simulink model "aircraft"  (R2018a)
settings: Solver=FixedStepAuto  StartTime=0.0  StopTime=10.0  FixedStep=0.02  RelTol=1e-3
model workspace (MAT data in the model file):
  Beta = 426.4352
  Gamma = 0.01
  Ka = 0.677
  Kf = -1.746
  Ki = -3.864
  Kq = 0.8156
  Md = -6.8847
  Mq = -0.6571
  Mw = -0.00592
  Sa = 0.005236
  Swg = 3
  Ta = 0.05
  Tal = 0.3959
  Ts = 0.1
  Uo = 689.4
  Vto = 690.4
  W1 = 2.971
  W2 = 4.144
  Wa = 10
  Zd = -63.9979
  Zw = -0.6385
  a = 2.5348
  b = 64.13
  cmdgain = 0.0349095447273
  g = 32.2
undefined symbols (not defined in the file): a_max, a_min, adva_max, adva_min, x_ini, x_max, x_min
libraries: simulink x2
settings Model: TunableVars=a_max,a_min,adva_max,adva_min,x_ini,x_max,x_min  TunableVarsStorageClass=Auto,Auto,Auto,Auto,Auto,Auto,Auto  TunableVarsTypeQualifier=,,,,,,  OrderedModelArguments=off  Creator=hjzsj  LastModifiedBy=Jet
settings DataIOCC: ReturnWorkspaceOutputs=on
settings OptimizationCC: DefaultParameterBehavior=Inlined  UseDivisionForNetSlopeComputation=on  UseFloatMulNetSlope=on  PassReuseOutputArgsAs=Individual arguments  NoFixptDivByZeroProtection=on  EfficientFloat2IntCast=on  LifeSpan=1  OptimizeBlockOrder=speed  DifferentSizesBufferReuse=on
settings DebuggingCC: ParameterTunabilityLossMsg=error
settings HardwareCC: ProdLongLongMode=on
settings SFSimCC: SimUseLocalCustomCode=on  MATLABDynamicMemAlloc=off
settings RTWCC: SystemTargetFile=ert.tlc  GenCodeOnly=on  TemplateMakefile=ert_default_tmf  PostCodeGenCommand=mat2json  RTWUseLocalCustomCode=on  TargetLang=C++
settings CodeAppCC: ForceParamTrailComments=on  IgnoreCustomStorageClasses=off  OperatorAnnotations=on  SimulinkDataObjDesc=on  SFDataObjDesc=on  CustomSymbolStrGlobalVar=rt$N$M  CustomSymbolStrType=$N$M  CustomSymbolStrFcn=$N$M$F  CustomSymbolStrMacro=$N$M  InsertBlockDesc=on
settings ERTTargetCC: TargetLangStandard=C++03 (ISO)  GenerateSampleERTMain=on  CombineSignalStateStructs=on  MultiInstanceERTCode=on  CodeInterfacePackaging=C++ class  SupportComplex=off  SupportContinuousTime=on  InlinedParameterPlacement=NonHierarchical  RootIOFormat=Structure reference  ERTCustomFileTemplate=example_file_process.tlc  ERTFilePackagingFormat=CompactWithDataFile

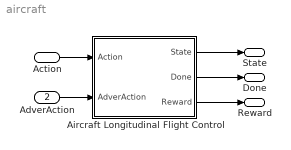
== system aircraft ==
  Action : Inport
  AdverAction : Inport  Port=2
  Aircraft Longitudinal Flight Control : Subsystem
  State : Outport  VectorParamsAs1DForOutWhenUnconnected=on
  Done : Outport  Port=2  VectorParamsAs1DForOutWhenUnconnected=on
  Reward : Outport  Port=3  VectorParamsAs1DForOutWhenUnconnected=on
  wires:
  Aircraft Longitudinal Flight Control/1(State) -> State/1
  Aircraft Longitudinal Flight Control/2(Done) -> Done/1
  Action/1 -> Aircraft Longitudinal Flight Control/1(Action)
  Aircraft Longitudinal Flight Control/3(Reward) -> Reward/1
  AdverAction/1 -> Aircraft Longitudinal Flight Control/2(AdverAction)

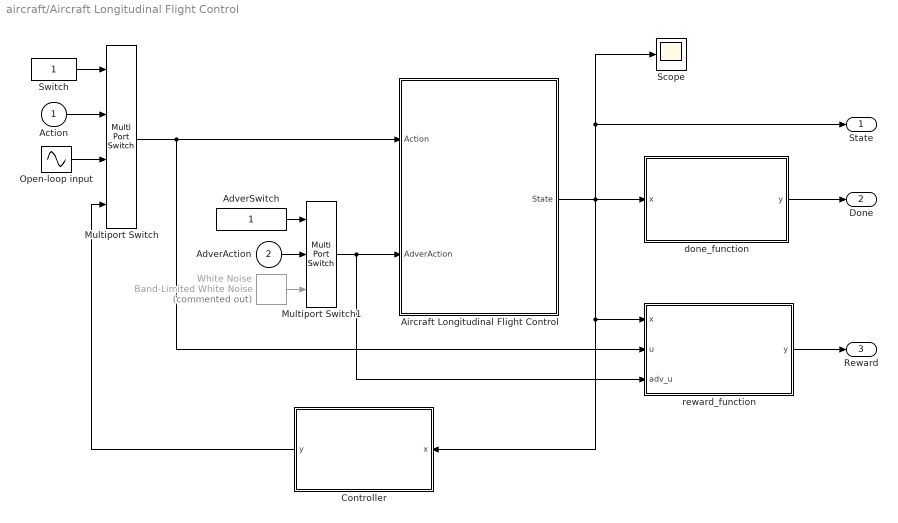
== system aircraft/Aircraft Longitudinal Flight Control ==
  Action : Inport
  AdverAction : Inport  Port=2
  AdverSwitch : Constant
  Aircraft Longitudinal Flight Control : Subsystem
  Controller : MATLAB Function  TreatAsAtomicUnit=on
  Multiport Switch : MultiPortSwitch
  Multiport Switch1 : MultiPortSwitch  Inputs=2
  Open-loop input : Sin  SampleTime=0
  Scope : Scope
  Switch : Constant
  White Noise : simulink/Sources/Band-Limited White Noise  Commented=on  Cov=[0.5]  Ts=0.02  seed=[23341]
  done_function : MATLAB Function  TreatAsAtomicUnit=on
  reward_function : MATLAB Function  TreatAsAtomicUnit=on
  State : Outport  VectorParamsAs1DForOutWhenUnconnected=on
  Done : Outport  Port=2  VectorParamsAs1DForOutWhenUnconnected=on
  Reward : Outport  Port=3  VectorParamsAs1DForOutWhenUnconnected=on
  wires:
  Aircraft Longitudinal Flight Control/1(State) -> Controller/1(x), reward_function/1(x), Scope/1, State/1, done_function/1(x)
  reward_function/1(y) -> Reward/1
  Open-loop input/1 -> Multiport Switch/3
  done_function/1(y) -> Done/1
  Switch/1 -> Multiport Switch/1
  Multiport Switch/1 -> reward_function/2(u), Aircraft Longitudinal Flight Control/1(Action)
  Action/1 -> Multiport Switch/2
  Controller/1(y) -> Multiport Switch/4
  Multiport Switch1/1 -> reward_function/3(adv_u), Aircraft Longitudinal Flight Control/2(AdverAction)
  AdverSwitch/1 -> Multiport Switch1/1
  White Noise/1 -> Multiport Switch1/3
  AdverAction/1 -> Multiport Switch1/2

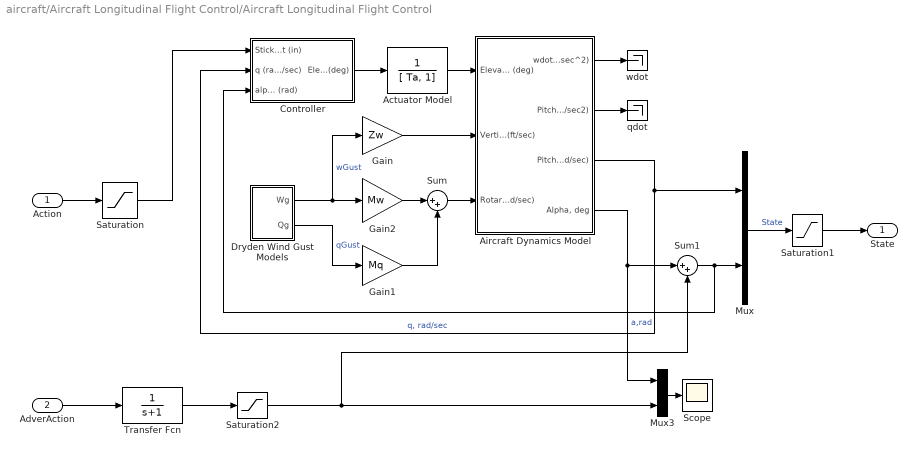
== system aircraft/Aircraft Longitudinal Flight Control/Aircraft Longitudinal Flight Control ==
  Action : Inport
  AdverAction : Inport  Port=2
  Actuator Model : TransferFcn  Denominator=[ Ta, 1]
  Aircraft Dynamics Model : Subsystem
      mask Display:
      | port_label('input',1,'\delta_{e}, deg','texmode','on');
      | port_label('input',2,'wGust, ft/sec','texmode','on');
      | port_label('input',3,'qGust, rad/sec','texmode','on');
      | port_label('output',1,'wdot, ft/sec^2','texmode','on');
      | port_label('output',2,'qdot, rad/sec^{2}','texmode','on');
      | port_label('output',3,'q, rad/sec','texmode','on');
      | port_label('output',4,'\alpha, rad','texmode','on');
  Controller : Subsystem
      mask Display:
      | port_label('input',1,'Stick, in','texmode','on');
      | port_label('input',3,'\alpha, rad','texmode','on');
      | port_label('input',2,'q, rad/sec','texmode','on');
      | port_label('output',1,'\deltacmd, deg','texmode','on');
  Dryden Wind Gust Models : Subsystem
      mask Display:
      | port_label('output',1,'wg','texmode','on');
      | port_label('output',2,'qg','texmode','on');
  Gain : Gain  Gain=Zw  SaturateOnIntegerOverflow=on  OutDataTypeStr=Inherit: Same as input  ParamDataTypeStr=Inherit: Same as input
  Gain1 : Gain  Gain=Mq  SaturateOnIntegerOverflow=on  OutDataTypeStr=Inherit: Same as input  ParamDataTypeStr=Inherit: Same as input
  Gain2 : Gain  Gain=Mw  SaturateOnIntegerOverflow=on  OutDataTypeStr=Inherit: Same as input  ParamDataTypeStr=Inherit: Same as input
  Mux : Mux  Inputs=2
  Mux3 : Mux  Inputs=2
  Saturation : Saturate  UpperLimit=a_max  LowerLimit=a_min
  Saturation1 : Saturate  UpperLimit=x_max  LowerLimit=x_min
  Saturation2 : Saturate  UpperLimit=adva_max  LowerLimit=adva_min
  Scope : Scope
  Sum : Sum  Inputs=|++  SaturateOnIntegerOverflow=on  InputSameDT=on  OutDataTypeStr=Inherit: Same as first input
  Sum1 : Sum  Inputs=|++
  Transfer Fcn : TransferFcn  Denominator=[1 1]
  qdot : Terminator
  wdot : Terminator
  State : Outport  VectorParamsAs1DForOutWhenUnconnected=on
  wires:
  Actuator Model/1 -> Aircraft Dynamics Model/1(Elevator Deflection d (deg))
  Dryden Wind Gust Models/1(Wg) -> Gain2/1, Gain/1  "wGust"
  Aircraft Dynamics Model/1(wdot (ft/sec^2)) -> wdot/1
  Saturation/1 -> Controller/1(Stick Input (in))
  Aircraft Dynamics Model/2(Pitch Accel qdot (rad/sec2)) -> qdot/1
  Gain2/1 -> Sum/1
  Controller/1(Elevator Command (deg)) -> Actuator Model/1
  Dryden Wind Gust Models/2(Qg) -> Gain1/1  "qGust"
  Gain1/1 -> Sum/2
  Gain/1 -> Aircraft Dynamics Model/2(Vertical Gust wGust (ft/sec))
  Sum/1 -> Aircraft Dynamics Model/3(Rotary Gust qGust (rad/sec))
  Aircraft Dynamics Model/3(Pitch Rate q (rad/sec)) -> Controller/2(q (rad/sec)), Mux/1  "q, rad/sec"
  Aircraft Dynamics Model/4("Alpha, deg") -> Mux3/1, Sum1/1  "a,rad"
  Action/1 -> Saturation/1
  Saturation1/1 -> State/1
  Mux/1 -> Saturation1/1  "State"
  Transfer Fcn/1 -> Saturation2/1
  Mux3/1 -> Scope/1
  AdverAction/1 -> Transfer Fcn/1
  Saturation2/1 -> Sum1/2, Mux3/2
  Sum1/1 -> Controller/3(alpha (rad)), Mux/2

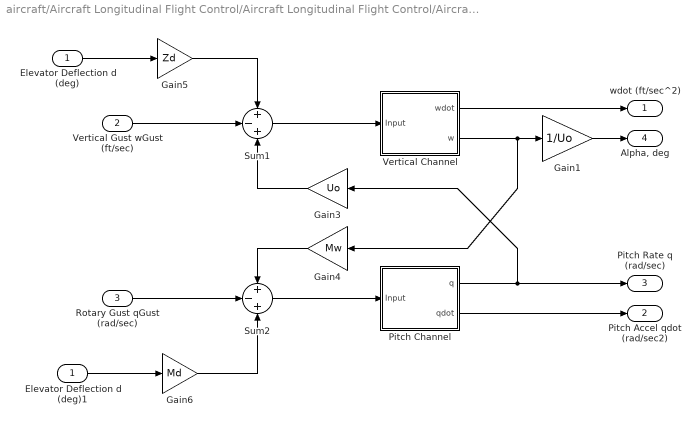
== system aircraft/Aircraft Longitudinal Flight Control/Aircraft Longitudinal Flight Control/Aircraft Dynamics Model ==
  Elevator Deflection d (deg) : Inport
  Vertical Gust wGust (ft/sec) : Inport  Port=2
  Rotary Gust qGust (rad/sec) : Inport  Port=3
  Elevator Deflection d (deg)1 : InportShadow
  Gain1 : Gain  Gain=1/Uo  SaturateOnIntegerOverflow=on  OutDataTypeStr=Inherit: Same as input  ParamDataTypeStr=Inherit: Same as input
  Gain3 : Gain  Gain=Uo  SaturateOnIntegerOverflow=on  OutDataTypeStr=Inherit: Same as input  ParamDataTypeStr=Inherit: Same as input
  Gain4 : Gain  Gain=Mw  SaturateOnIntegerOverflow=on  OutDataTypeStr=Inherit: Same as input  ParamDataTypeStr=Inherit: Same as input
  Gain5 : Gain  Gain=Zd  SaturateOnIntegerOverflow=on  OutDataTypeStr=Inherit: Same as input  ParamDataTypeStr=Inherit: Same as input
  Gain6 : Gain  Gain=Md  SaturateOnIntegerOverflow=on  OutDataTypeStr=Inherit: Same as input  ParamDataTypeStr=Inherit: Same as input
  Pitch Channel : Subsystem
  Sum1 : Sum  Inputs=+-+  SaturateOnIntegerOverflow=on  InputSameDT=on  OutDataTypeStr=Inherit: Same as first input
  Sum2 : Sum  Inputs=+-+  SaturateOnIntegerOverflow=on  InputSameDT=on  OutDataTypeStr=Inherit: Same as first input
  Vertical Channel : Subsystem
  wdot (ft/sec^2) : Outport  InitialOutput=0
  Pitch Accel qdot (rad/sec2) : Outport  Port=2  InitialOutput=0
  Pitch Rate q (rad/sec) : Outport  Port=3  InitialOutput=0
  "Alpha, deg" : Outport  Port=4  InitialOutput=0
  wires:
  Vertical Channel/2(w) -> Gain4/1, Gain1/1
  Pitch Channel/1(q) -> Pitch Rate q (rad/sec)/1, Gain3/1
  Gain6/1 -> Sum2/3
  Gain5/1 -> Sum1/1
  Gain3/1 -> Sum1/3
  Rotary Gust qGust (rad/sec)/1 -> Sum2/2
  Sum2/1 -> Pitch Channel/1(Input)
  Sum1/1 -> Vertical Channel/1(Input)
  Gain4/1 -> Sum2/1
  Vertical Gust wGust (ft/sec)/1 -> Sum1/2
  Elevator Deflection d (deg)/1 -> Gain5/1
  Elevator Deflection d (deg)1/1 -> Gain6/1
  Gain1/1 -> "Alpha, deg"/1
  Vertical Channel/1(wdot) -> wdot (ft/sec^2)/1
  Pitch Channel/2(qdot) -> Pitch Accel qdot (rad/sec2)/1

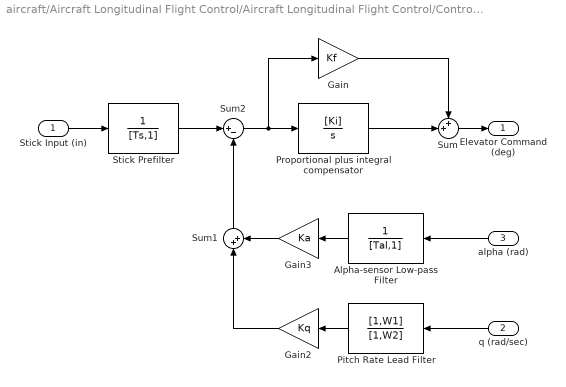
== system aircraft/Aircraft Longitudinal Flight Control/Aircraft Longitudinal Flight Control/Controller ==
  Stick Input (in) : Inport
  q (rad/sec) : Inport  Port=2
  alpha (rad) : Inport  Port=3
  Alpha-sensor Low-pass Filter : TransferFcn  Denominator=[Tal,1]
  Gain : Gain  Gain=Kf  SaturateOnIntegerOverflow=on  OutDataTypeStr=Inherit: Same as input  ParamDataTypeStr=Inherit: Same as input
  Gain2 : Gain  Gain=Kq  SaturateOnIntegerOverflow=on  OutDataTypeStr=Inherit: Same as input  ParamDataTypeStr=Inherit: Same as input
  Gain3 : Gain  Gain=Ka  SaturateOnIntegerOverflow=on  OutDataTypeStr=Inherit: Same as input  ParamDataTypeStr=Inherit: Same as input
  Pitch Rate Lead Filter : TransferFcn  Numerator=[1,W1]  Denominator=[1,W2]
  Proportional plus integral compensator : TransferFcn  Numerator=[Ki]  Denominator=[1,0]
  Stick Prefilter : TransferFcn  Denominator=[Ts,1]
  Sum : Sum  Inputs=++|  SaturateOnIntegerOverflow=on  InputSameDT=on  OutDataTypeStr=Inherit: Same as first input
  Sum1 : Sum  Inputs=|++  SaturateOnIntegerOverflow=on  InputSameDT=on  OutDataTypeStr=Inherit: Same as first input
  Sum2 : Sum  Inputs=|+-  SaturateOnIntegerOverflow=on  InputSameDT=on  OutDataTypeStr=Inherit: Same as first input
  Elevator Command (deg) : Outport  InitialOutput=0
  wires:
  Sum2/1 -> Proportional plus integral compensator/1, Gain/1
  Gain/1 -> Sum/1
  Proportional plus integral compensator/1 -> Sum/2
  Stick Prefilter/1 -> Sum2/1
  Sum/1 -> Elevator Command (deg)/1
  Gain2/1 -> Sum1/1
  Gain3/1 -> Sum1/2
  Sum1/1 -> Sum2/2
  Pitch Rate Lead Filter/1 -> Gain2/1
  q (rad/sec)/1 -> Pitch Rate Lead Filter/1
  Alpha-sensor Low-pass Filter/1 -> Gain3/1
  alpha (rad)/1 -> Alpha-sensor Low-pass Filter/1
  Stick Input (in)/1 -> Stick Prefilter/1

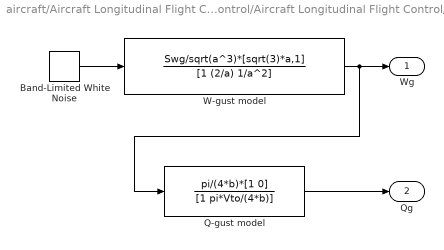
== system aircraft/Aircraft Longitudinal Flight Control/Aircraft Longitudinal Flight Control/Dryden Wind Gust Models ==
  Band-Limited White Noise : simulink/Sources/Band-Limited White Noise  Cov=1  Ts=0.1  seed=[23341]
  Q-gust model : TransferFcn  Numerator=pi/(4*b)*[1 0]  Denominator=[1 pi*Vto/(4*b)]
  W-gust model : TransferFcn  Numerator=Swg/sqrt(a^3)*[sqrt(3)*a,1]  Denominator=[1 (2/a) 1/a^2]
  Wg : Outport  InitialOutput=0
  Qg : Outport  Port=2  InitialOutput=0
  wires:
  Band-Limited White Noise/1 -> W-gust model/1
  Q-gust model/1 -> Qg/1
  W-gust model/1 -> Wg/1, Q-gust model/1

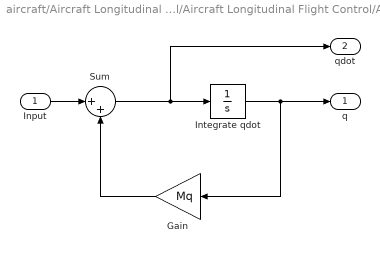
== system aircraft/Aircraft Longitudinal Flight Control/Aircraft Longitudinal Flight Control/Aircraft Dynamics Model/Pitch Channel ==
  Input : Inport
  Gain : Gain  Gain=Mq  SaturateOnIntegerOverflow=on  OutDataTypeStr=Inherit: Same as input  ParamDataTypeStr=Inherit: Same as input
  Integrate qdot : Integrator  InitialCondition=x_ini(2)
  Sum : Sum  Inputs=|++  SaturateOnIntegerOverflow=on  InputSameDT=on  OutDataTypeStr=Inherit: Same as first input
  q : Outport  InitialOutput=0
  qdot : Outport  Port=2  InitialOutput=0
  wires:
  Sum/1 -> qdot/1, Integrate qdot/1
  Integrate qdot/1 -> Gain/1, q/1
  Gain/1 -> Sum/2
  Input/1 -> Sum/1

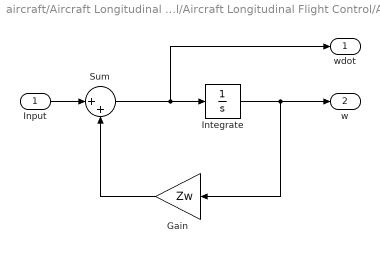
== system aircraft/Aircraft Longitudinal Flight Control/Aircraft Longitudinal Flight Control/Aircraft Dynamics Model/Vertical Channel ==
  Input : Inport
  Gain : Gain  Gain=Zw  SaturateOnIntegerOverflow=on  OutDataTypeStr=Inherit: Same as input  ParamDataTypeStr=Inherit: Same as input
  Integrate : Integrator  InitialCondition=x_ini(1)
  Sum : Sum  Inputs=|++  SaturateOnIntegerOverflow=on  InputSameDT=on  OutDataTypeStr=Inherit: Same as first input
  wdot : Outport  InitialOutput=0
  w : Outport  Port=2  InitialOutput=0
  wires:
  Input/1 -> Sum/1
  Gain/1 -> Sum/2
  Integrate/1 -> w/1, Gain/1
  Sum/1 -> Integrate/1, wdot/1

== matlab function aircraft/Aircraft Longitudinal Flight Control/Controller ==
  data: x input; y output
function y = fcn(x)
done = (abs(x(1))>0.75);
y = done;

== matlab function aircraft/Aircraft Longitudinal Flight Control/done_function ==
  data: x input; y output
function y = fcn(x)
done = (abs(x(1))>0.75);
y = done;

== matlab function aircraft/Aircraft Longitudinal Flight Control/reward_function ==
  data: x input; u input; y output; adv_u input
function y = fcn(x, u, adv_u)

y = -(x(2)-0)^2 - u^2;
